simulink model "Week2_Problem2"  (R2020a)
settings: Solver=VariableStepAuto  StartTime=0.0  StopTime=10.0  RelTol=1e-3
values from neighbouring files (symbols this model uses):
  be = 2.0    [Problem2data.sldd]
  bv = 1.0    [Problem2data.sldd]
  Ie = 1.0    [Problem2data.sldd]
  Iv = 5.0    [Problem2data.sldd]
settings Model: DataDictionary=Problem2data.sldd  Creator=tnradm  LastModifiedBy=tnradm

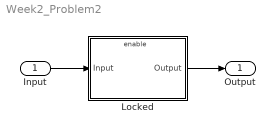
== system Week2_Problem2 ==
  Input : Inport
  Locked : Subsystem
  Output : Outport
  wires:
  Input/1 -> Locked/1(Input)
  Locked/1(Output) -> Output/1

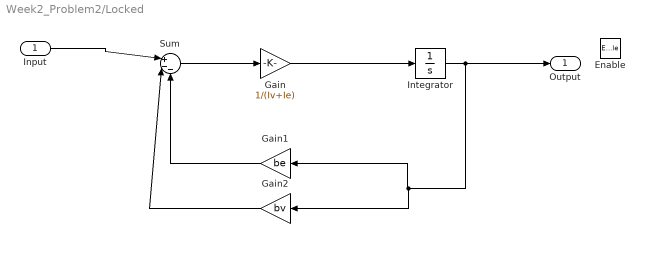
== system Week2_Problem2/Locked ==
  Input : Inport
  Enable : EnablePort
  Gain : Gain  Gain=1/(Iv+Ie)
  Gain1 : Gain  Gain=be
  Gain2 : Gain  Gain=bv
  Integrator : Integrator
  Sum : Sum  Inputs=|+--
  Output : Outport
  wires:
  Gain/1 -> Integrator/1
  Gain1/1 -> Sum/3
  Integrator/1 -> Output/1, Gain1/1, Gain2/1
  Input/1 -> Sum/1
  Gain2/1 -> Sum/2
  Sum/1 -> Gain/1
